simulink model "PmsmSmo"  (R2016a)
settings: Solver=ode45  StartTime=0.0  StopTime=0.2  RelTol=1e-3
libraries: powerlib x6, dsparch4 x2, simulink x1
settings Model: Creator=lovejing  LastModifiedBy=Administrator
settings SolverCC: ZeroCrossAlgorithm=Adaptive
settings DataIOCC: LimitDataPoints=on  SaveFormat=Array  SignalLoggingSaveFormat=ModelDataLogs
settings OptimizationCC: ExpressionDepthLimit=2147483647
settings DebuggingCC: UnderspecifiedInitializationDetection=Classic  MergeDetectMultiDrivingBlocksExec=none  SolverPrmCheckMsg=warning  FcnCallInpInsideContextMsg=UseLocalSettings  StateNameClashWarn=warning
settings HardwareCC: ProdBitPerPointer=32  ProdLargestAtomicFloat=None  ProdIntDivRoundTo=Undefined  ProdEndianess=Unspecified  ProdWordSize=32  ProdHWDeviceType=32-bit Generic
settings ModelReferenceCC: PropagateSignalLabelsOutOfModel=off
settings GRTTargetCC: CombineOutputUpdateFcns=off  GRTInterface=on
settings ConfigComp: CovModelRefEnable=Off  CovSFcnEnable=off

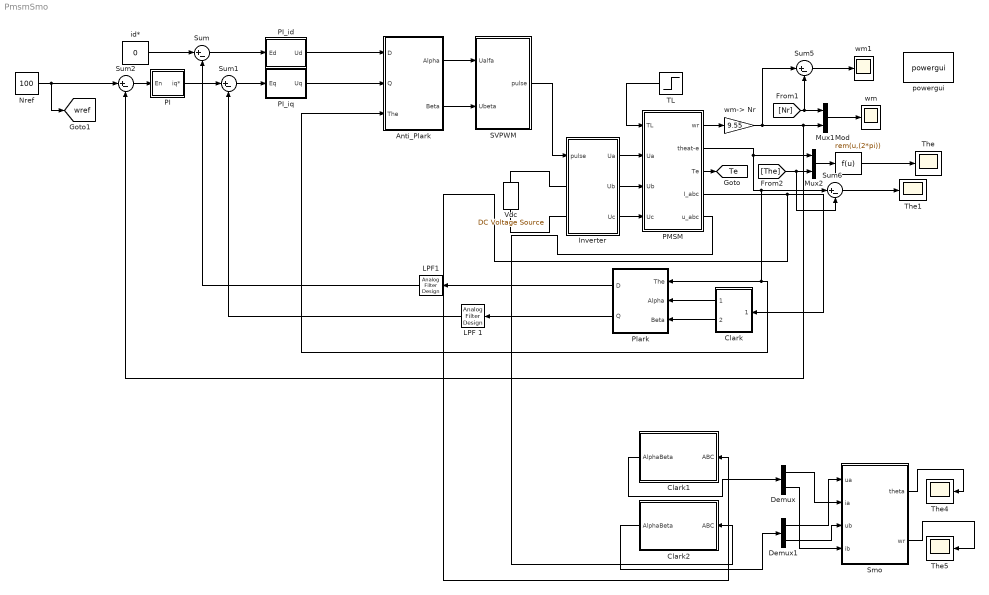
== system PmsmSmo ==
  Anti_Plark : Subsystem
  Clark : Subsystem
  Clark1 : Subsystem
  Clark2 : Subsystem
  Demux : Demux  Outputs=2
  Demux1 : Demux  Outputs=2
  Inverter : Subsystem
  LPF 1 : dsparch4/Analog Filter Design  method=Butterworth  filttype=Lowpass  N=1  Wlo=942  Whi=80  Rp=2  Rs=40
  LPF1 : dsparch4/Analog Filter Design  method=Butterworth  filttype=Lowpass  N=1  Wlo=942  Whi=80  Rp=2  Rs=40
  Mod : Fcn  Expr=rem(u,(2*pi))
  Mux1 : Mux  Inputs=2
  Mux2 : Mux  Inputs=2
  Nref : Constant  Value=100
  PI : Subsystem  mask{Knp=0.4, Kni=2}
  PI_id : Subsystem  mask{Kip=40, Kii=1}
  PI_iq : Subsystem  mask{Kip=40, Kii=1}
  PMSM : Subsystem  mask{Ld=0.0052, R=0.33, Lq=0.0052, kf=0.646, p=2, F=0, J=0.008}
  Plark : Subsystem
  SVPWM : Subsystem
  Smo : Subsystem  mask{R=0.33, L=0.0052, K1=0.1}
  Sum{,1..2,5..6} (5 alike) : Sum  Inputs=|+-
  TL : Step  Time=0.05  After=0  SampleTime=0
  The{,1,4..5} (4 alike) : Scope
  "Vdc " : powerlib/Electrical Sources/DC Voltage Source  Amplitude=311  Measurements=None
  id* : Constant  Value=0
  powergui : powerlib/powergui  Priority=1  SimulationMode=Continuous  SolverType=Tustin/Backward Euler (TBE)  SampleTime=50e-6  frequency=60  SPID=off  DisableSnubberDevices=off  DisableRonSwitches=off  DisableVfSwitches=off  SwTol=0  DisplayEquations=off  Interpol=off  ExternalGateDelay=off  methode=off  Ts=100  FunctionMessages=off  echomessages=off  HookPort=off  EnableUseOfTLC=off  x0status=blocks  frequencyindice=0  Pbase=100e6  ErrMax=1e-4  Iterations=50  UnitsV=kV  UnitsW=MW  buscounter=0  RestoreLinks=warning  ResistiveCurrentMeasurement=off  Frange=[0:2:500]  Ylog=off  Xlog=on  ShowGrid=off  save=off  variable=ZData  structure=0  ZoomFFT=off  StartTime=0.0  cycles=1  DisplayStyle=1  fundamental=60  FreqAxis=off  MaxFrequency=1000  frequencyindicesteady=1  RmsSteady=1  display=off
  wm : Scope
  wm-> Nr : Gain  Gain=9.55
  wm1 : Scope
  tag scope: Te=global, wref=global
  wires:
  Clark/2(Beta) -> Plark/3(Beta)
  id*/1 -> Sum/1
  Plark/1(D) -> LPF1/1
  Sum/1 -> PI_id/1(Ed)
  Plark/2(Q) -> LPF 1/1
  Nref/1 -> [wref], Sum2/1
  Sum2/1 -> PI/1(En)
  Sum1/1 -> PI_iq/1(Eq)
  PI/1(iq*) -> Sum1/1
  PI_iq/1(Uq) -> Anti_Plark/2(Q)
  SVPWM/1(pulse) -> Inverter/1(pulse)
  Anti_Plark/1(Alpha) -> SVPWM/1(Ualfa)
  Anti_Plark/2(Beta) -> SVPWM/2(Ubeta)
  Sum6/1 -> The1/1
  Inverter/2(Ub) -> PMSM/3(Ub)
  Inverter/3(Uc) -> PMSM/4(Uc)
  Inverter/1(Ua) -> PMSM/2(Ua)
  PMSM/1(wr) -> wm-> Nr/1
  TL/1 -> PMSM/1(TL)
  Mux1/1 -> wm/1
  PMSM/3(Te) -> [Te]
  [Nr] -> Sum5/2, Mux1/1
  [The] -> Mux2/2, Sum6/2
  Mux2/1 -> Mod/1
  Sum5/1 -> wm1/1
  PI_id/1(Ud) -> Anti_Plark/1(D)
  PMSM/2(theat-e) -> Mux2/1, Plark/1(The), Anti_Plark/3(The), Sum6/1
  wm-> Nr/1 -> Sum5/1, Sum2/2, Mux1/2
  Mod/1 -> The/1
  Clark/1(Alpha) -> Plark/2(Alpha)
  Clark1/1(AlphaBeta) -> Demux/1
  PMSM/4(I_abc) -> Clark1/1(ABC), Clark/1(ABC)
  Clark2/1(AlphaBeta) -> Demux1/1
  PMSM/5(u_abc) -> Clark2/1(ABC)
  Demux/1 -> Smo/2(ia)
  Demux/2 -> Smo/4(ib)
  Demux1/1 -> Smo/1(ua)
  Demux1/2 -> Smo/3(ub)
  Smo/1(theta) -> The4/1
  Smo/2(wr) -> The5/1
  LPF 1/1 -> Sum1/2
  LPF1/1 -> Sum/2
  connections:
  Inverter/LConn2 -- "Vdc "/LConn1
  Inverter/LConn1 -- "Vdc "/RConn1

== system PmsmSmo/Anti_Plark ==
  D : Inport
  Q : Inport  Port=2
  The : Inport  Port=3
  Mux : Mux  Inputs=3
  alpha : Fcn  Expr=u(1)*cos(u(3))-u(2)*sin(u(3))
  beta : Fcn  Expr=u(1)*sin(u(3))+u(2)*cos(u(3))
  Alpha : Outport
  Beta : Outport  Port=2
  wires:
  alpha/1 -> Alpha/1
  Q/1 -> Mux/2
  The/1 -> Mux/3
  D/1 -> Mux/1
  Mux/1 -> beta/1, alpha/1
  beta/1 -> Beta/1

== system PmsmSmo/Clark ==
  ABC : Inport
  alpha : Fcn  Expr=(u(1)-0.5*(u(2)+u(3)))*2/3
  beta : Fcn  Expr=sqrt(3)/2*(u(2)-u(3))*2/3
  Alpha : Outport
  Beta : Outport  Port=2
  wires:
  alpha/1 -> Alpha/1
  ABC/1 -> beta/1, alpha/1
  beta/1 -> Beta/1

== system PmsmSmo/Clark1 ==
  ABC : Inport
  Mux : Mux  Inputs=2
  alpha : Fcn  Expr=(u(1)-0.5*(u(2)+u(3)))*2/3
  beta : Fcn  Expr=sqrt(3)/2*(u(2)-u(3))*2/3
  AlphaBeta : Outport
  wires:
  ABC/1 -> alpha/1, beta/1
  alpha/1 -> Mux/1
  beta/1 -> Mux/2
  Mux/1 -> AlphaBeta/1

== system PmsmSmo/Clark2 ==
  ABC : Inport
  Mux : Mux  Inputs=2
  alpha : Fcn  Expr=(u(1)-0.5*(u(2)+u(3)))*2/3
  beta : Fcn  Expr=sqrt(3)/2*(u(2)-u(3))*2/3
  AlphaBeta : Outport
  wires:
  Mux/1 -> AlphaBeta/1
  beta/1 -> Mux/2
  alpha/1 -> Mux/1
  ABC/1 -> beta/1, alpha/1

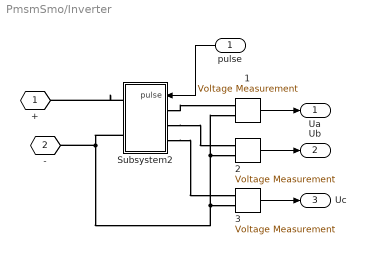
== system PmsmSmo/Inverter ==
  pulse : Inport
  1 : powerlib/Measurements/Voltage Measurement  PhasorSimulation=off  OutputType=Complex  PSBequivalent=0
  2 : powerlib/Measurements/Voltage Measurement  PhasorSimulation=off  OutputType=Complex  PSBequivalent=0
  3 : powerlib/Measurements/Voltage Measurement  PhasorSimulation=off  OutputType=Complex  PSBequivalent=0
  Subsystem2 : Subsystem
  + : PMIOPort  Tag=PMCPort  Port=1  Side=Left
  - : PMIOPort  Tag=PMCPort  Port=2  Side=Left
  Ua : Outport
  Ub : Outport  Port=2
  Uc : Outport  Port=3
  wires:
  3/1 -> Uc/1
  2/1 -> Ub/1
  1/1 -> Ua/1
  pulse/1 -> Subsystem2/1(pulse)
  connections:
  Subsystem2/LConn1 -- 1/LConn1
  -/RConn1 -- Subsystem2/RConn2 -- 3/LConn2 -- 2/LConn2 -- 1/LConn2
  Subsystem2/LConn2 -- 2/LConn1
  Subsystem2/LConn3 -- 3/LConn1
  Subsystem2/RConn1 -- +/RConn1

== system PmsmSmo/PI ==
  En : Inport
  Gain : Gain  Gain=Kni
  Gain1 : Gain  Gain=Knp
  Integrator : Integrator
  Saturation : Saturate  UpperLimit=50  LowerLimit=-50
  Subtract : Sum
  iq* : Outport
  wires:
  En/1 -> Gain/1, Gain1/1
  Gain/1 -> Integrator/1
  Integrator/1 -> Subtract/1
  Gain1/1 -> Subtract/2
  Subtract/1 -> Saturation/1
  Saturation/1 -> iq*/1

== system PmsmSmo/PI_id ==
  Ed : Inport
  Gain : Gain  Gain=Kii
  Gain1 : Gain  Gain=Kip
  Integrator : Integrator
  Saturation : Saturate  UpperLimit=10  LowerLimit=-10
  Subtract : Sum
  Ud : Outport
  wires:
  Ed/1 -> Gain/1, Gain1/1
  Gain/1 -> Integrator/1
  Integrator/1 -> Subtract/1
  Gain1/1 -> Subtract/2
  Subtract/1 -> Saturation/1
  Saturation/1 -> Ud/1

== system PmsmSmo/PI_iq ==
  Eq : Inport
  Gain : Gain  Gain=Kii
  Gain1 : Gain  Gain=Kip
  Integrator : Integrator
  Saturation : Saturate  UpperLimit=100  LowerLimit=-100
  Subtract : Sum
  Uq : Outport
  wires:
  Eq/1 -> Gain/1, Gain1/1
  Gain/1 -> Integrator/1
  Integrator/1 -> Subtract/1
  Gain1/1 -> Subtract/2
  Subtract/1 -> Saturation/1
  Saturation/1 -> Uq/1

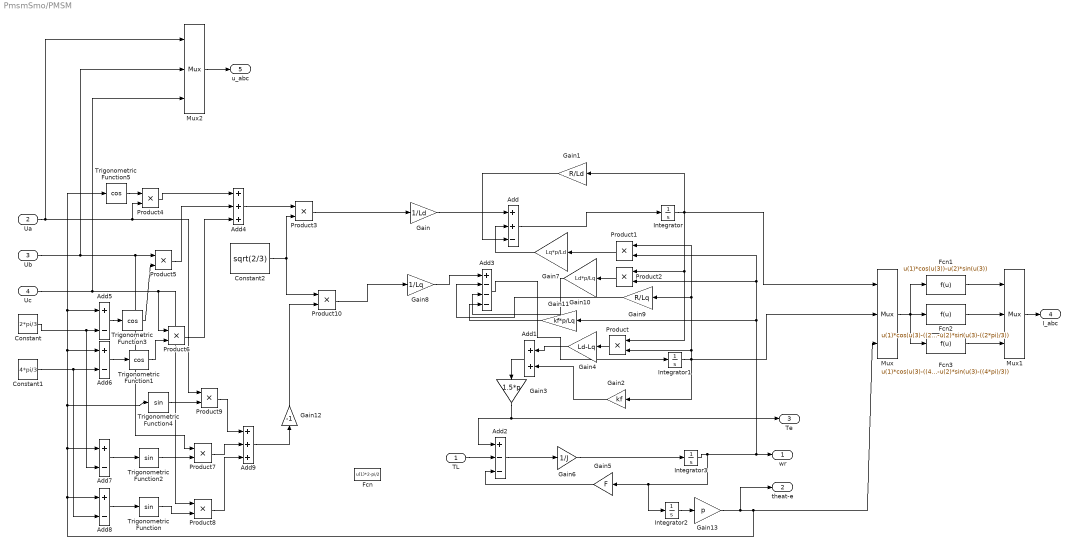
== system PmsmSmo/PMSM ==
  TL : Inport
  Ua : Inport  Port=2
  Ub : Inport  Port=3
  Uc : Inport  Port=4
  Add : Sum  Inputs=++-
  Add1 : Sum
  Add2 : Sum  Inputs=+--
  Add3 : Sum  Inputs=+---
  Add4 : Sum  Inputs=+++
  Add{5..8} (4 alike) : Sum  Inputs=+-
  Add9 : Sum  Inputs=+++
  Constant : Constant  Value=2*pi/3
  Constant1 : Constant  Value=4*pi/3
  Constant2 : Constant  Value=sqrt(2/3)
  Fcn : Fcn  Expr=u(1)*2-pi/2
  Fcn1 : Fcn  Expr=u(1)*cos(u(3))-u(2)*sin(u(3))
  Fcn2 : Fcn  Expr=u(1)*cos(u(3)-((2*pi)/3))-u(2)*sin(u(3)-((2*pi)/3))
  Fcn3 : Fcn  Expr=u(1)*cos(u(3)-((4*pi)/3))-u(2)*sin(u(3)-((4*pi)/3))
  Gain : Gain  Gain=1/Ld
  Gain1 : Gain  Gain=R/Ld
  Gain10 : Gain  Gain=Ld*p/Lq
  Gain11 : Gain  Gain=kf*p/Lq
  Gain12 : Gain  Gain=-1
  Gain13 : Gain  Gain=p
  Gain2 : Gain  Gain=kf
  Gain3 : Gain  Gain=1.5*p
  Gain4 : Gain  Gain=Ld-Lq
  Gain5 : Gain  Gain=F
  Gain6 : Gain  Gain=1/J
  Gain7 : Gain  Gain=Lq*p/Ld
  Gain8 : Gain  Gain=1/Lq
  Gain9 : Gain  Gain=R/Lq
  Integrator{,1..3} (4 alike) : Integrator
  Mux : Mux  Inputs=3
  Mux1 : Mux  Inputs=3
  Mux2 : Mux  Inputs=3
  Product{,1..10} (11 alike) : Product  RndMeth=Zero
  Trigonometric Function : Trigonometry
  Trigonometric Function1 : Trigonometry  Operator=cos
  Trigonometric Function2 : Trigonometry
  Trigonometric Function3 : Trigonometry  Operator=cos
  Trigonometric Function4 : Trigonometry
  Trigonometric Function5 : Trigonometry  Operator=cos
  wr : Outport
  theat-e : Outport  Port=2
  Te : Outport  Port=3
  I_abc : Outport  Port=4
  u_abc : Outport  Port=5
  wires:
  Add3/1 -> Integrator1/1
  Gain11/1 -> Add3/4
  Gain10/1 -> Add3/3
  Product2/1 -> Gain10/1
  Gain9/1 -> Add3/2
  Gain8/1 -> Add3/1
  Add/1 -> Integrator/1
  Gain7/1 -> Add/2
  Product1/1 -> Gain7/1
  Gain6/1 -> Integrator3/1
  Add2/1 -> Gain6/1
  Gain5/1 -> Add2/3
  TL/1 -> Add2/2
  Integrator3/1 -> wr/1, Product1/2, Product2/2, Gain11/1, Gain5/1, Integrator2/1
  Gain3/1 -> Add2/1, Te/1
  Add1/1 -> Gain3/1
  Gain2/1 -> Add1/2
  Gain4/1 -> Add1/1
  Product/1 -> Gain4/1
  Gain1/1 -> Add/3
  Integrator1/1 -> Product/2, Product1/1, Gain9/1, Gain2/1, Mux/2
  Integrator/1 -> Gain1/1, Product/1, Product2/1, Mux/1
  Gain/1 -> Add/1
  Constant2/1 -> Product3/2, Product10/1
  Add4/1 -> Product3/1
  Product3/1 -> Gain/1
  Constant/1 -> Add5/2, Add7/2
  Add5/1 -> Trigonometric Function3/1
  Constant1/1 -> Add6/2, Add8/2
  Add6/1 -> Trigonometric Function1/1
  Trigonometric Function5/1 -> Product4/1
  Ua/1 -> Mux2/1, Product4/2, Product9/1
  Product4/1 -> Add4/1
  Ub/1 -> Mux2/2, Product5/1, Product7/1
  Trigonometric Function3/1 -> Product5/2
  Product5/1 -> Add4/2
  Uc/1 -> Mux2/3, Product6/1, Product8/1
  Trigonometric Function1/1 -> Product6/2
  Product6/1 -> Add4/3
  Add7/1 -> Trigonometric Function2/1
  Add8/1 -> Trigonometric Function/1
  Trigonometric Function2/1 -> Product7/2
  Trigonometric Function/1 -> Product8/2
  Trigonometric Function4/1 -> Product9/2
  Product9/1 -> Add9/1
  Product7/1 -> Add9/2
  Product8/1 -> Add9/3
  Add9/1 -> Gain12/1
  Gain12/1 -> Product10/2
  Product10/1 -> Gain8/1
  Gain13/1 -> Add8/1, Add7/1, Trigonometric Function5/1, Add5/1, Add6/1, Trigonometric Function4/1, Mux/3, theat-e/1
  Fcn3/1 -> Mux1/3
  Fcn2/1 -> Mux1/2
  Fcn1/1 -> Mux1/1
  Mux/1 -> Fcn2/1, Fcn1/1, Fcn3/1
  Mux1/1 -> I_abc/1
  Integrator2/1 -> Gain13/1
  Mux2/1 -> u_abc/1

== system PmsmSmo/Plark ==
  The : Inport
  Alpha : Inport  Port=2
  Beta : Inport  Port=3
  Mux : Mux  Inputs=3
  d : Fcn  Expr=u(1)*cos(u(3))+u(2)*sin(u(3))
  q : Fcn  Expr=-u(1)*sin(u(3))+u(2)*cos(u(3))
  D : Outport
  Q : Outport  Port=2
  wires:
  d/1 -> D/1
  Beta/1 -> Mux/2
  The/1 -> Mux/3
  Alpha/1 -> Mux/1
  Mux/1 -> q/1, d/1
  q/1 -> Q/1

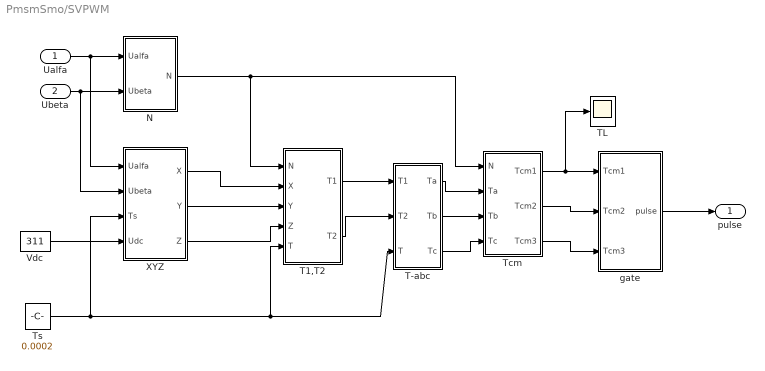
== system PmsmSmo/SVPWM ==
  Ualfa : Inport
  Ubeta : Inport  Port=2
  N : Subsystem
  T-abc : Subsystem
  T1,T2 : Subsystem
  TL : Scope
  Tcm : Subsystem
  Ts : Constant  Value=0.0002  SampleTime=-1
  Vdc : Constant  Value=311
  XYZ : Subsystem
  gate : Subsystem
  pulse : Outport
  wires:
  Tcm/1(Tcm1) -> gate/1(Tcm1), TL/1
  T-abc/2(Tb) -> Tcm/3(Tb)
  T-abc/1(Ta) -> Tcm/2(Ta)
  T-abc/3(Tc) -> Tcm/4(Tc)
  T1,T2/1(T1) -> T-abc/1(T1)
  T1,T2/2(T2) -> T-abc/2(T2)
  XYZ/2(Y) -> T1,T2/3(Y)
  XYZ/1(X) -> T1,T2/2(X)
  XYZ/3(Z) -> T1,T2/4(Z)
  N/1(N) -> T1,T2/1(N), Tcm/1(N)
  Ts/1 -> T1,T2/5(T), T-abc/3(T), XYZ/3(Ts)
  gate/1(pulse) -> pulse/1
  Ualfa/1 -> N/1(Ualfa), XYZ/1(Ualfa)
  Ubeta/1 -> N/2(Ubeta), XYZ/2(Ubeta)
  Vdc/1 -> XYZ/4(Udc)
  Tcm/2(Tcm2) -> gate/2(Tcm2)
  Tcm/3(Tcm3) -> gate/3(Tcm3)

== system PmsmSmo/Smo ==
  ua : Inport
  ia : Inport  Port=2
  ub : Inport  Port=3
  ib : Inport  Port=4
  PLL : Subsystem
  反电动势滑模观测 : Subsystem
  theta : Outport
  wr : Outport  Port=2
  wires:
  PLL/1(theta) -> theta/1
  PLL/2(wr) -> wr/1
  ua/1 -> 反电动势滑模观测/1(In1)
  ia/1 -> 反电动势滑模观测/2(In2)
  ub/1 -> 反电动势滑模观测/3(In3)
  ib/1 -> 反电动势滑模观测/4(In4)
  反电动势滑模观测/1(Out1) -> PLL/1(ea)
  反电动势滑模观测/2(Out2) -> PLL/2(eb)

== system PmsmSmo/Inverter/Subsystem2 ==
  pulse : Inport
  Universal Bridge : powerlib/Power Electronics/Universal Bridge  Arms=3  SnubberResistance=1e5  SnubberCapacitance=inf  Device=IGBT / Diodes  Ron=1e-3  Lon=0  ForwardVoltages="[  0  0  ]"  ForwardVoltage=0  GTOparameters=[ 10e-6 , 20e-6 ]  IGBTparameters=[ 1e-6 , 2e-6 ]  Measurements=None  Measurements_2=None  converterType=Rectifier
  Ua : PMIOPort  Tag=PMCPort  Port=1  Side=Left
  Ub : PMIOPort  Tag=PMCPort  Port=2  Side=Left
  Uc : PMIOPort  Tag=PMCPort  Port=3  Side=Left
  + : PMIOPort  Tag=PMCPort  Port=4  Side=Right
  - : PMIOPort  Tag=PMCPort  Port=5  Side=Right
  wires:
  pulse/1 -> Universal Bridge/1
  connections:
  Universal Bridge/LConn1 -- Ua/RConn1
  Universal Bridge/LConn2 -- Ub/RConn1
  Universal Bridge/LConn3 -- Uc/RConn1
  +/RConn1 -- Universal Bridge/RConn1
  -/RConn1 -- Universal Bridge/RConn2

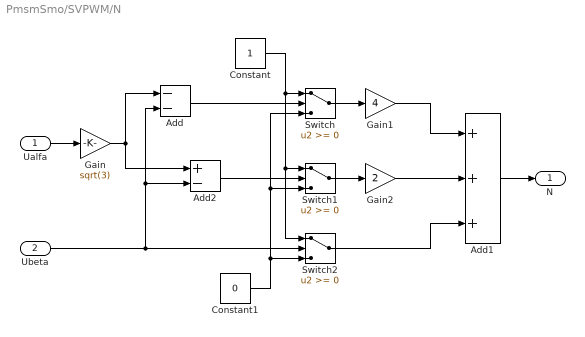
== system PmsmSmo/SVPWM/N ==
  Ualfa : Inport
  Ubeta : Inport  Port=2
  Add : Sum  Inputs=--
  Add1 : Sum  Inputs=+++
  Add2 : Sum  Inputs=+-
  Constant : Constant
  Constant1 : Constant  Value=0
  Gain : Gain  Gain=sqrt(3)
  Gain1 : Gain  Gain=4
  Gain2 : Gain  Gain=2
  Switch : Switch
  Switch1 : Switch
  Switch2 : Switch
  N : Outport
  wires:
  Ualfa/1 -> Gain/1
  Add1/1 -> N/1
  Switch/1 -> Gain1/1
  Add/1 -> Switch/2
  Gain/1 -> Add/1, Add2/1
  Ubeta/1 -> Switch2/2, Add/2, Add2/2
  Gain1/1 -> Add1/1
  Switch2/1 -> Add1/3
  Add2/1 -> Switch1/2
  Switch1/1 -> Gain2/1
  Gain2/1 -> Add1/2
  Constant/1 -> Switch2/1, Switch1/1, Switch/1
  Constant1/1 -> Switch/3, Switch1/3, Switch2/3

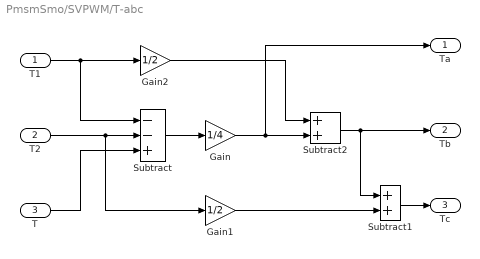
== system PmsmSmo/SVPWM/T-abc ==
  T1 : Inport
  T2 : Inport  Port=2
  T : Inport  Port=3
  Gain : Gain  Gain=1/4
  Gain1 : Gain  Gain=1/2
  Gain2 : Gain  Gain=1/2
  Subtract : Sum  Inputs=--+
  Subtract1 : Sum
  Subtract2 : Sum
  Ta : Outport
  Tb : Outport  Port=2
  Tc : Outport  Port=3
  wires:
  T2/1 -> Subtract/2, Gain1/1
  T1/1 -> Subtract/1, Gain2/1
  T/1 -> Subtract/3
  Subtract/1 -> Gain/1
  Gain/1 -> Ta/1, Subtract2/2
  Gain2/1 -> Subtract2/1
  Subtract2/1 -> Tb/1, Subtract1/1
  Subtract1/1 -> Tc/1
  Gain1/1 -> Subtract1/2

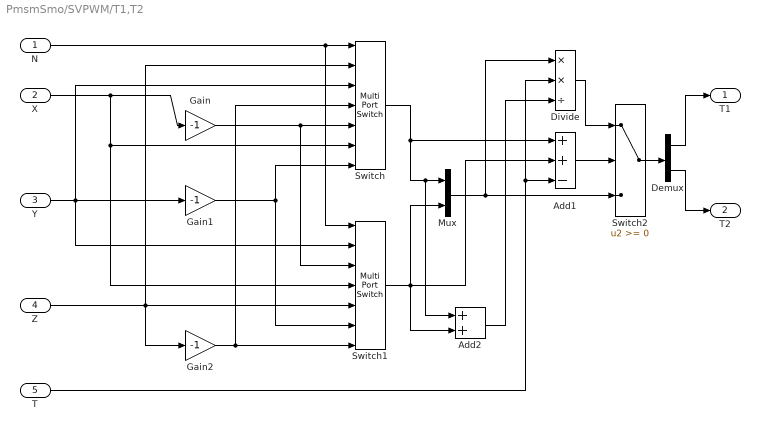
== system PmsmSmo/SVPWM/T1,T2 ==
  N : Inport
  X : Inport  Port=2
  Y : Inport  Port=3
  Z : Inport  Port=4
  T : Inport  Port=5
  Add1 : Sum  Inputs=++-
  Add2 : Sum
  Demux : Demux  Outputs=2
  Divide : Product  Inputs=**/
  Gain : Gain  Gain=-1
  Gain1 : Gain  Gain=-1
  Gain2 : Gain  Gain=-1
  Mux : Mux  Inputs=2
  Switch : MultiPortSwitch  Inputs=6
  Switch1 : MultiPortSwitch  Inputs=6
  Switch2 : Switch
  T1 : Outport
  T2 : Outport  Port=2
  wires:
  Y/1 -> Switch/3, Gain1/1, Switch1/2
  Z/1 -> Switch/2, Switch1/5, Gain2/1
  X/1 -> Gain/1, Switch1/4, Switch/6
  Gain/1 -> Switch/5, Switch1/3
  Gain2/1 -> Switch/4, Switch1/7
  Gain1/1 -> Switch1/6, Switch/7
  Switch/1 -> Add1/1, Mux/1, Add2/1
  Switch1/1 -> Mux/2, Add1/2, Add2/2
  Mux/1 -> Divide/1, Switch2/3
  Switch2/1 -> Demux/1
  Demux/1 -> T1/1
  Demux/2 -> T2/1
  Add1/1 -> Switch2/2
  T/1 -> Add1/3, Divide/2
  Divide/1 -> Switch2/1
  Add2/1 -> Divide/3
  N/1 -> Switch/1, Switch1/1

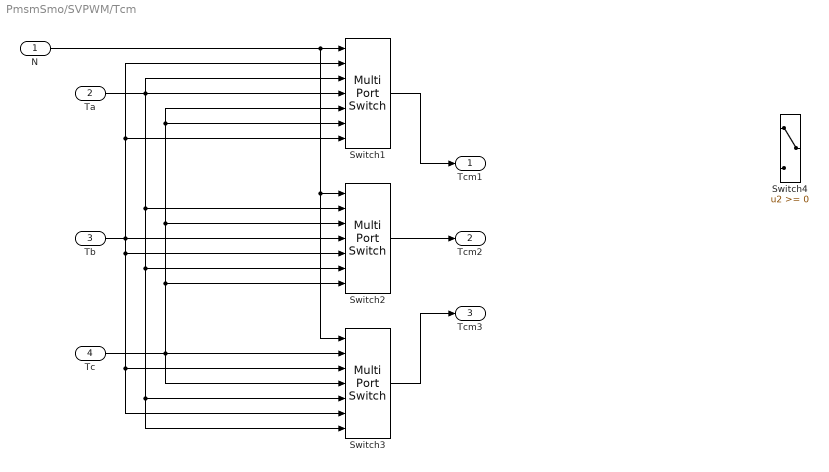
== system PmsmSmo/SVPWM/Tcm ==
  N : Inport
  Ta : Inport  Port=2
  Tb : Inport  Port=3
  Tc : Inport  Port=4
  Switch1 : MultiPortSwitch  Inputs=6
  Switch2 : MultiPortSwitch  Inputs=6
  Switch3 : MultiPortSwitch  Inputs=6
  Switch4 : Switch
  Tcm1 : Outport
  Tcm2 : Outport  Port=2
  Tcm3 : Outport  Port=3
  wires:
  Switch2/1 -> Tcm2/1
  Switch3/1 -> Tcm3/1
  Switch1/1 -> Tcm1/1
  Tb/1 -> Switch2/4, Switch2/5, Switch3/3, Switch3/6, Switch1/2, Switch1/7
  Tc/1 -> Switch3/2, Switch3/4, Switch2/3, Switch1/5, Switch1/6, Switch2/7
  Ta/1 -> Switch1/4, Switch1/3, Switch2/2, Switch2/6, Switch3/5, Switch3/7
  N/1 -> Switch1/1, Switch2/1, Switch3/1

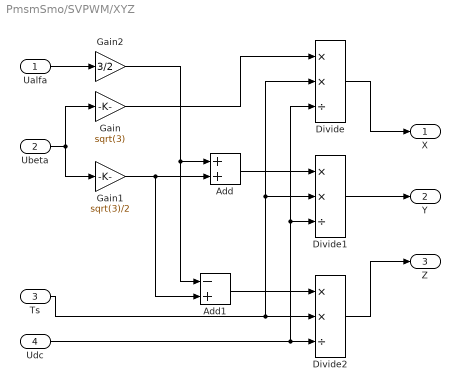
== system PmsmSmo/SVPWM/XYZ ==
  Ualfa : Inport
  Ubeta : Inport  Port=2
  Ts : Inport  Port=3
  Udc : Inport  Port=4
  Add : Sum
  Add1 : Sum  Inputs=-+
  Divide : Product  Inputs=**/
  Divide1 : Product  Inputs=**/
  Divide2 : Product  Inputs=**/
  Gain : Gain  Gain=sqrt(3)
  Gain1 : Gain  Gain=sqrt(3)/2
  Gain2 : Gain  Gain=3/2
  X : Outport
  Y : Outport  Port=2
  Z : Outport  Port=3
  wires:
  Divide1/1 -> Y/1
  Divide/1 -> X/1
  Divide2/1 -> Z/1
  Ts/1 -> Divide2/2, Divide1/2, Divide/2
  Udc/1 -> Divide2/3, Divide1/3, Divide/3
  Ubeta/1 -> Gain/1, Gain1/1
  Ualfa/1 -> Gain2/1
  Gain/1 -> Divide/1
  Add/1 -> Divide1/1
  Gain1/1 -> Add/2, Add1/2
  Gain2/1 -> Add1/1, Add/1
  Add1/1 -> Divide2/1

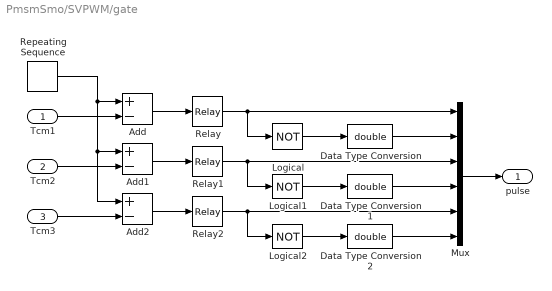
== system PmsmSmo/SVPWM/gate ==
  Tcm1 : Inport
  Tcm2 : Inport  Port=2
  Tcm3 : Inport  Port=3
  Add : Sum  Inputs=+-
  Add1 : Sum  Inputs=+-
  Add2 : Sum  Inputs=+-
  Data Type Conversion : DataTypeConversion  OutDataTypeStr=double
  Data Type Conversion1 : DataTypeConversion  OutDataTypeStr=double
  Data Type Conversion2 : DataTypeConversion  OutDataTypeStr=double
  Logical : Logic  Operator=NOT  AllPortsSameDT=off  OutDataTypeStr=boolean
  Logical1 : Logic  Operator=NOT  AllPortsSameDT=off  OutDataTypeStr=boolean
  Logical2 : Logic  Operator=NOT  AllPortsSameDT=off  OutDataTypeStr=boolean
  Mux : Mux  Inputs=6
  Relay : Relay
  Relay1 : Relay
  Relay2 : Relay
  Repeating Sequence : simulink/Sources/Repeating Sequence  rep_seq_t=[0 0.00005 0.0001]  rep_seq_y=[0 0.0001 0]
  pulse : Outport
  wires:
  Tcm1/1 -> Add/2
  Tcm2/1 -> Add1/2
  Tcm3/1 -> Add2/2
  Repeating Sequence/1 -> Add2/1, Add1/1, Add/1
  Add2/1 -> Relay2/1
  Add1/1 -> Relay1/1
  Add/1 -> Relay/1
  Relay/1 -> Mux/1, Logical/1
  Relay1/1 -> Mux/3, Logical1/1
  Relay2/1 -> Mux/5, Logical2/1
  Data Type Conversion/1 -> Mux/2
  Logical/1 -> Data Type Conversion/1
  Data Type Conversion1/1 -> Mux/4
  Logical1/1 -> Data Type Conversion1/1
  Data Type Conversion2/1 -> Mux/6
  Logical2/1 -> Data Type Conversion2/1
  Mux/1 -> pulse/1

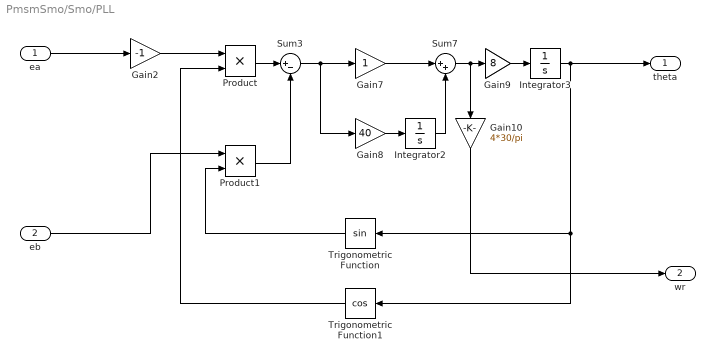
== system PmsmSmo/Smo/PLL ==
  ea : Inport
  eb : Inport  Port=2
  Gain10 : Gain  Gain=4*30/pi
  Gain2 : Gain  Gain=-1
  Gain7 : Gain
  Gain8 : Gain  Gain=40
  Gain9 : Gain  Gain=8
  Integrator2 : Integrator
  Integrator3 : Integrator
  Product : Product  RndMeth=Zero
  Product1 : Product  RndMeth=Zero
  Sum3 : Sum  Inputs=|+-
  Sum7 : Sum  Inputs=|++
  Trigonometric Function : Trigonometry
  Trigonometric Function1 : Trigonometry  Operator=cos
  theta : Outport
  wr : Outport  Port=2
  wires:
  eb/1 -> Product1/1
  ea/1 -> Gain2/1
  Gain2/1 -> Product/1
  Product/1 -> Sum3/1
  Product1/1 -> Sum3/2
  Sum3/1 -> Gain7/1, Gain8/1
  Gain8/1 -> Integrator2/1
  Gain7/1 -> Sum7/1
  Integrator2/1 -> Sum7/2
  Sum7/1 -> Gain10/1, Gain9/1
  Trigonometric Function1/1 -> Product/2
  Trigonometric Function/1 -> Product1/2
  Integrator3/1 -> theta/1, Trigonometric Function/1, Trigonometric Function1/1
  Gain9/1 -> Integrator3/1
  Gain10/1 -> wr/1

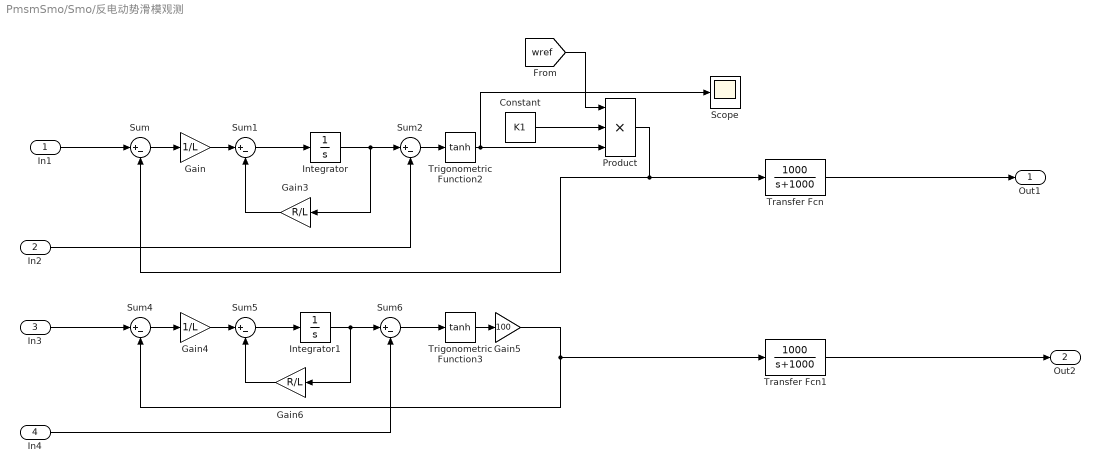
== system PmsmSmo/Smo/反电动势滑模观测 ==
  In1 : Inport
  In2 : Inport  Port=2
  In3 : Inport  Port=3
  In4 : Inport  Port=4
  Constant : Constant  Value=K1
  Gain : Gain  Gain=1/L
  Gain3 : Gain  Gain=R/L
  Gain4 : Gain  Gain=1/L
  Gain5 : Gain  Gain=100
  Gain6 : Gain  Gain=R/L
  Integrator : Integrator
  Integrator1 : Integrator
  Product : Product  Inputs=3
  Scope : Scope
  Sum{,1..2,4..6} (6 alike) : Sum  Inputs=|+-
  Transfer Fcn : TransferFcn  Numerator=[1000]  Denominator=[1 1000]
  Transfer Fcn1 : TransferFcn  Numerator=[1000]  Denominator=[1 1000]
  Trigonometric Function2 : Trigonometry  Operator=tanh
  Trigonometric Function3 : Trigonometry  Operator=tanh
  Out1 : Outport
  Out2 : Outport  Port=2
  wires:
  Sum/1 -> Gain/1
  Gain/1 -> Sum1/1
  Sum1/1 -> Integrator/1
  Integrator/1 -> Sum2/1, Gain3/1
  Gain3/1 -> Sum1/2
  Sum4/1 -> Gain4/1
  Gain4/1 -> Sum5/1
  Sum5/1 -> Integrator1/1
  Integrator1/1 -> Sum6/1, Gain6/1
  Sum6/1 -> Trigonometric Function3/1
  Gain6/1 -> Sum5/2
  In2/1 -> Sum2/2
  In3/1 -> Sum4/1
  In4/1 -> Sum6/2
  In1/1 -> Sum/1
  Trigonometric Function3/1 -> Gain5/1
  Trigonometric Function2/1 -> Product/3, Scope/1
  Sum2/1 -> Trigonometric Function2/1
  Product/1 -> Sum/2, Transfer Fcn/1
  Gain5/1 -> Transfer Fcn1/1, Sum4/2
  [wref] -> Product/1
  Constant/1 -> Product/2
  Transfer Fcn/1 -> Out1/1
  Transfer Fcn1/1 -> Out2/1
